simulink model "Load_Oserver"  (R2015a)
settings: Solver=ode4  StartTime=0.0  StopTime=0.1  FixedStep=1e-6  MaxStep=0.00001  MinStep=0.000001  RelTol=1e-3
libraries: powerlib x10, simulink x5, powerlib_meascontrol x3
settings Model: Creator=hp  LastModifiedBy=hp
settings SolverCC: ZeroCrossControl=DisableAll

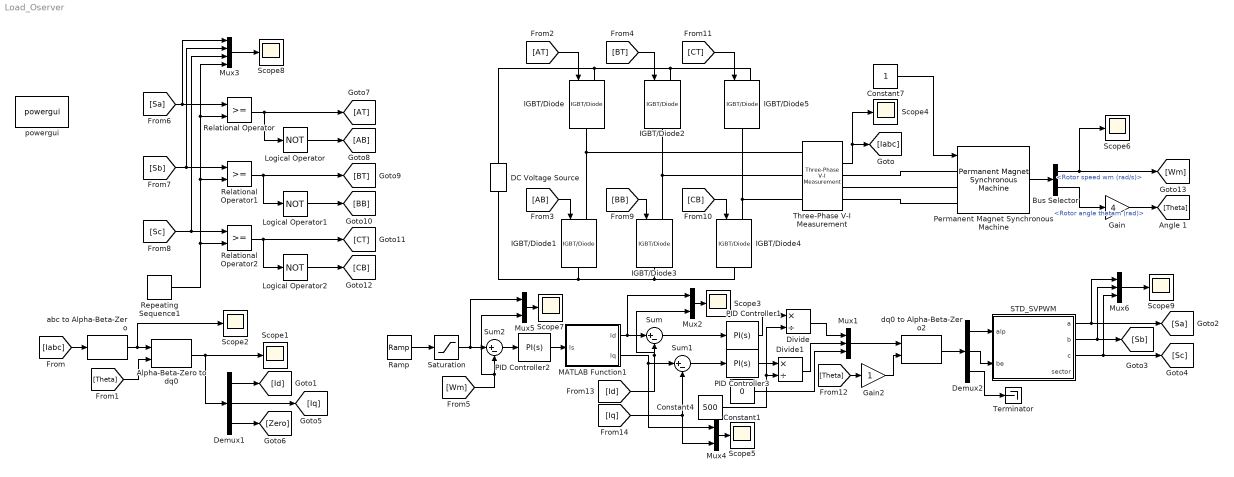
== system Load_Oserver ==
  Alpha-Beta-Zero to dq0 : powerlib_meascontrol/Transformations/Alpha-Beta-Zero to dq0  Alignment=Aligned with phase A axis
  Bus Selector : BusSelector  OutputSignals=Rotor speed wm (rad/s),Rotor angle thetam (rad)
  Constant1 : Constant  Value=0
  Constant4 : Constant  Value=500
  Constant7 : Constant
  DC Voltage Source : powerlib/Electrical Sources/DC Voltage Source  Amplitude=500  Measurements=None
  Demux1 : Demux  Outputs=3
  Demux2 : Demux  Outputs=3
  Divide : Product  Inputs=*/
  Divide1 : Product  Inputs=*/
  Gain : Gain  Gain=4
  Gain2 : Gain
  IGBT/Diode{,1..5} (6 alike) : powerlib/Power Electronics/IGBT//Diode  Ron=1e-3  Rs=1e5  Cs=inf  Measurements=off
  Logical Operator : Logic  Operator=NOT  Inputs=1  AllPortsSameDT=off  OutDataTypeStr=boolean
  Logical Operator1 : Logic  Operator=NOT  Inputs=1  AllPortsSameDT=off  OutDataTypeStr=boolean
  Logical Operator2 : Logic  Operator=NOT  Inputs=1  AllPortsSameDT=off  OutDataTypeStr=boolean
  MATLAB Function1 : MATLAB Function  TreatAsAtomicUnit=on
  Mux1 : Mux  Inputs=3
  Mux2 : Mux  Inputs=2
  Mux3 : Mux
  Mux4 : Mux  Inputs=2
  Mux5 : Mux  Inputs=2
  Mux6 : Mux  Inputs=3
  PID Controller1 : simulink/Continuous/PID Controller  Controller=PI  TimeDomain=Continuous-time  SampleTime=-1  IntegratorMethod=Forward Euler  FilterMethod=Forward Euler  Form=Parallel  UseFilter=on  ControllerParametersSource=internal  P=40  I=15000  D=0  N=100  InitialConditionSource=internal  InitialConditionForIntegrator=0  InitialConditionForFilter=0  ExternalReset=none  LimitOutput=off  UpperSaturationLimit=inf  LowerSaturationLimit=-inf  LinearizeAsGain=on  AntiWindupMode=none  Kb=1  TrackingMode=off  Kt=1  PParamMin=[]  PParamMax=[]  IParamMin=[]  IParamMax=[]  DParamMin=[]  DParamMax=[]  NParamMin=[]  NParamMax=[]  KbParamMin=[]  KbParamMax=[]  KtParamMin=[]  KtParamMax=[]  POutMin=[]  POutMax=[]  IOutMin=[]  IOutMax=[]  DOutMin=[]  DOutMax=[]  NOutMin=[]  NOutMax=[]  KbOutMin=[]  KbOutMax=[]  KtOutMin=[]  KtOutMax=[]  IntegratorOutMin=[]  IntegratorOutMax=[]  FilterOutMin=[]  FilterOutMax=[]  SumOutMin=[]  SumOutMax=[]  SumI1OutMin=[]  SumI1OutMax=[]  SumI2OutMin=[]  SumI2OutMax=[]  SumI3OutMin=[]  SumI3OutMax=[]  SumDOutMin=[]  SumDOutMax=[]  SaturationOutMin=[]  SaturationOutMax=[]  IntegratorContinuousStateAttributes=''  IntegratorStateMustResolveToSignalObject=off  IntegratorRTWStateStorageClass=Auto  FilterContinuousStateAttributes=''  FilterStateMustResolveToSignalObject=off  FilterRTWStateStorageClass=Auto  DifferentiatorICPrevScaledInput=0  DifferentiatorOutMin=[]  DifferentiatorOutMax=[]
  PID Controller2 : simulink/Continuous/PID Controller  Controller=PI  TimeDomain=Continuous-time  SampleTime=-1  IntegratorMethod=Forward Euler  FilterMethod=Forward Euler  Form=Parallel  UseFilter=on  ControllerParametersSource=internal  P=60  I=10000  D=0  N=100  InitialConditionSource=internal  InitialConditionForIntegrator=0  InitialConditionForFilter=0  ExternalReset=none  LimitOutput=off  UpperSaturationLimit=inf  LowerSaturationLimit=-inf  LinearizeAsGain=on  AntiWindupMode=none  Kb=1  TrackingMode=off  Kt=1  PParamMin=[]  PParamMax=[]  IParamMin=[]  IParamMax=[]  DParamMin=[]  DParamMax=[]  NParamMin=[]  NParamMax=[]  KbParamMin=[]  KbParamMax=[]  KtParamMin=[]  KtParamMax=[]  POutMin=[]  POutMax=[]  IOutMin=[]  IOutMax=[]  DOutMin=[]  DOutMax=[]  NOutMin=[]  NOutMax=[]  KbOutMin=[]  KbOutMax=[]  KtOutMin=[]  KtOutMax=[]  IntegratorOutMin=[]  IntegratorOutMax=[]  FilterOutMin=[]  FilterOutMax=[]  SumOutMin=[]  SumOutMax=[]  SumI1OutMin=[]  SumI1OutMax=[]  SumI2OutMin=[]  SumI2OutMax=[]  SumI3OutMin=[]  SumI3OutMax=[]  SumDOutMin=[]  SumDOutMax=[]  SaturationOutMin=[]  SaturationOutMax=[]  IntegratorContinuousStateAttributes=''  IntegratorStateMustResolveToSignalObject=off  IntegratorRTWStateStorageClass=Auto  FilterContinuousStateAttributes=''  FilterStateMustResolveToSignalObject=off  FilterRTWStateStorageClass=Auto  DifferentiatorICPrevScaledInput=0  DifferentiatorOutMin=[]  DifferentiatorOutMax=[]
  PID Controller3 : simulink/Continuous/PID Controller  Controller=PI  TimeDomain=Continuous-time  SampleTime=-1  IntegratorMethod=Forward Euler  FilterMethod=Forward Euler  Form=Parallel  UseFilter=on  ControllerParametersSource=internal  P=40  I=15000  D=0  N=100  InitialConditionSource=internal  InitialConditionForIntegrator=0  InitialConditionForFilter=0  ExternalReset=none  LimitOutput=off  UpperSaturationLimit=inf  LowerSaturationLimit=-inf  LinearizeAsGain=on  AntiWindupMode=none  Kb=1  TrackingMode=off  Kt=1  PParamMin=[]  PParamMax=[]  IParamMin=[]  IParamMax=[]  DParamMin=[]  DParamMax=[]  NParamMin=[]  NParamMax=[]  KbParamMin=[]  KbParamMax=[]  KtParamMin=[]  KtParamMax=[]  POutMin=[]  POutMax=[]  IOutMin=[]  IOutMax=[]  DOutMin=[]  DOutMax=[]  NOutMin=[]  NOutMax=[]  KbOutMin=[]  KbOutMax=[]  KtOutMin=[]  KtOutMax=[]  IntegratorOutMin=[]  IntegratorOutMax=[]  FilterOutMin=[]  FilterOutMax=[]  SumOutMin=[]  SumOutMax=[]  SumI1OutMin=[]  SumI1OutMax=[]  SumI2OutMin=[]  SumI2OutMax=[]  SumI3OutMin=[]  SumI3OutMax=[]  SumDOutMin=[]  SumDOutMax=[]  SaturationOutMin=[]  SaturationOutMax=[]  IntegratorContinuousStateAttributes=''  IntegratorStateMustResolveToSignalObject=off  IntegratorRTWStateStorageClass=Auto  FilterContinuousStateAttributes=''  FilterStateMustResolveToSignalObject=off  FilterRTWStateStorageClass=Auto  DifferentiatorICPrevScaledInput=0  DifferentiatorOutMin=[]  DifferentiatorOutMax=[]
  Permanent Magnet Synchronous Machine : powerlib/Machines/Permanent Magnet Synchronous Machine  NbPhases=3  FluxDistribution=Sinusoidal  RotorType=Salient-pole  MechanicalLoad=Torque Tm  PresetModel=No  ShowDetailedParameters=on  MeasurementBus=off  Resistance=2.07  Inductance=8.5e-3  dqInductances=[30.0e-3,2.5e-3]  La=5e-3  MachineConstant=Voltage Constant (V_peak L-L / krpm)  Flux=0.075808  VoltageCst=55  TorqueCst=0.45485  Flat=120  Mechanical=[0.00027 0.004924 4 0]  PolePairs=2  InitialConditions=[0,0, 0,0]  InitialConditions5ph=[0 0 0 0 0 0]  TsPowergui=0  TsBlock=-1  RefAngle=Aligned with phase A axis (original Park)
  Ramp : simulink/Sources/Ramp  slope=10000  start=0  X0=0
  Relational Operator : RelationalOperator  OutDataTypeStr=boolean
  Relational Operator1 : RelationalOperator  OutDataTypeStr=boolean
  Relational Operator2 : RelationalOperator  OutDataTypeStr=boolean
  Repeating Sequence1 : simulink/Sources/Repeating Sequence  rep_seq_t=[0 0.5 1]/10000  rep_seq_y=[0 1 0]
  STD_SVPWM : MATLAB Function  TreatAsAtomicUnit=on
  Saturation : Saturate  UpperLimit=300  LowerLimit=-300
  Scope{1..9} (9 alike) : Scope
      Scope1 settings: YMin=-22.5  YMax=7.5
      Scope2 settings: YMin=-1  YMax=1.75  SaveName=ScopeData2
      Scope3 settings: TimeRange=0.08752399999999999  YMin=-2  YMax=14
      Scope4 settings: YMin=-15  YMax=15  SaveName=ScopeData5
      Scope5 settings: YMin=-54  YMax=55  SaveName=ScopeData3
      Scope6 settings: YMin=-100  YMax=100  SaveName=ScopeData6
      Scope7 settings: TimeRange=0.1  YMax=500  SaveName=ScopeData4
      Scope8 settings: YMin=0  YMax=1  SaveName=ScopeData7
      Scope9 settings: YMin=0.225  YMax=0.775  SaveName=ScopeData8
  Sum : Sum  Inputs=|+-
  Sum1 : Sum  Inputs=|+-
  Sum2 : Sum  Inputs=|+-
  Terminator : Terminator
  Three-Phase V-I Measurement : powerlib/Measurements/Three-Phase V-I Measurement  VoltageMeasurement=phase-to-phase  SetLabelV=off  LabelV=Vabc  Vpu=off  VpuLL=off  CurrentMeasurement=yes  SetLabelI=off  LabelI=Iabc  Ipu=off  Pbase=100e6  Vbase=500e3  OutputType=Complex  PhasorSimulation=off  PSBequivalent=0
  abc to Alpha-Beta-Zero : powerlib_meascontrol/Transformations/abc to Alpha-Beta-Zero
  dq0 to Alpha-Beta-Zero2 : powerlib_meascontrol/Transformations/dq0 to Alpha-Beta-Zero  Alignment=Aligned with phase A axis
  powergui : powerlib/powergui  Priority=1  SimulationMode=Discrete  SolverType=Tustin/Backward Euler (TBE)  SampleTime=1e-6  frequency=60  SPID=off  DisableSnubberDevices=off  DisableRonSwitches=off  DisableVfSwitches=off  SwTol=0  DisplayEquations=off  Interpol=off  methode=off  Ts=100  FunctionMessages=off  echomessages=off  HookPort=off  EnableUseOfTLC=off  x0status=blocks  frequencyindice=0  Pbase=100e6  ErrMax=1e-4  Iterations=50  UnitsV=kV  UnitsW=MW  buscounter=0  RestoreLinks=warning  ResistiveCurrentMeasurement=off  Frange=[0:2:500]  Ylog=off  Xlog=on  ShowGrid=off  save=off  variable=ZData  structure=0  ZoomFFT=off  StartTime=0.0  cycles=1  DisplayStyle=1  fundamental=60  FreqAxis=off  MaxFrequency=1000  frequencyindicesteady=1  RmsSteady=1  display=off
  wires:
  STD_SVPWM/1(a) -> Mux6/1, [Sa]
  STD_SVPWM/2(b) -> Mux6/2, [Sb]
  STD_SVPWM/3(c) -> Mux6/3, [Sc]
  Three-Phase V-I Measurement/2 -> Scope4/1, [Iabc]
  [Iabc] -> abc to Alpha-Beta-Zero/1
  Alpha-Beta-Zero to dq0/1 -> Demux1/1, Scope1/1
  abc to Alpha-Beta-Zero/1 -> Scope2/1, Alpha-Beta-Zero to dq0/1
  [Theta] -> Alpha-Beta-Zero to dq0/2
  Demux1/1 -> [Id]
  Demux1/2 -> [Iq]
  Demux1/3 -> [Zero]
  [Sa] -> Mux3/1, Relational Operator/1
  Repeating Sequence1/1 -> Relational Operator2/2, Mux3/4, Relational Operator/2, Relational Operator1/2
  [Sb] -> Mux3/2, Relational Operator1/1
  [Sc] -> Mux3/3, Relational Operator2/1
  Relational Operator/1 -> Logical Operator/1, [AT]
  Logical Operator/1 -> [AB]
  Relational Operator1/1 -> Logical Operator1/1, [BT]
  Logical Operator1/1 -> [BB]
  Relational Operator2/1 -> Logical Operator2/1, [CT]
  Logical Operator2/1 -> [CB]
  [AT] -> IGBT/Diode/1
  [AB] -> IGBT/Diode1/1
  [BT] -> IGBT/Diode2/1
  [BB] -> IGBT/Diode3/1
  [CB] -> IGBT/Diode4/1
  [CT] -> IGBT/Diode5/1
  dq0 to Alpha-Beta-Zero2/1 -> Demux2/1
  Demux2/1 -> STD_SVPWM/1(alp)
  Demux2/2 -> STD_SVPWM/2(be)
  Demux2/3 -> Terminator/1
  [Theta] -> Gain2/1
  Gain2/1 -> dq0 to Alpha-Beta-Zero2/2
  Mux1/1 -> dq0 to Alpha-Beta-Zero2/1
  Constant1/1 -> Mux1/3
  Sum/1 -> PID Controller1/1
  Sum1/1 -> PID Controller3/1
  Mux2/1 -> Scope3/1
  [Iq] -> Mux4/2, Sum1/2
  Mux4/1 -> Scope5/1
  [Id] -> Mux2/2, Sum/2
  Constant7/1 -> Permanent Magnet Synchronous Machine/1
  Permanent Magnet Synchronous Machine/1 -> Bus Selector/1
  Bus Selector/1 -> [Wm], Scope6/1  "<Rotor speed wm (rad/s)>"
  Gain/1 -> [Theta]
  Bus Selector/2 -> Gain/1  "<Rotor angle thetam (rad)>"
  Divide/1 -> Mux1/1
  PID Controller3/1 -> Divide1/1
  Divide1/1 -> Mux1/2
  PID Controller1/1 -> Divide/1
  Constant4/1 -> Divide/2, Divide1/2
  Mux3/1 -> Scope8/1
  MATLAB Function1/1(Id) -> Mux2/1, Sum/1
  Sum2/1 -> PID Controller2/1
  Saturation/1 -> Mux5/1, Sum2/1
  Ramp/1 -> Saturation/1
  Mux5/1 -> Scope7/1
  [Wm] -> Mux5/2, Sum2/2
  Mux6/1 -> Scope9/1
  MATLAB Function1/2(Iq) -> Mux4/1, Sum1/1
  PID Controller2/1 -> MATLAB Function1/1(Is)
  connections:
  Three-Phase V-I Measurement/RConn1 -- Permanent Magnet Synchronous Machine/LConn1
  Three-Phase V-I Measurement/RConn2 -- Permanent Magnet Synchronous Machine/LConn2
  Three-Phase V-I Measurement/RConn3 -- Permanent Magnet Synchronous Machine/LConn3
  IGBT/Diode/RConn1 -- IGBT/Diode1/LConn1 -- Three-Phase V-I Measurement/LConn1
  IGBT/Diode2/RConn1 -- Three-Phase V-I Measurement/LConn2 -- IGBT/Diode3/LConn1
  IGBT/Diode5/RConn1 -- Three-Phase V-I Measurement/LConn3 -- IGBT/Diode4/LConn1
  IGBT/Diode1/RConn1 -- DC Voltage Source/LConn1 -- IGBT/Diode3/RConn1 -- IGBT/Diode4/RConn1
  IGBT/Diode/LConn1 -- DC Voltage Source/RConn1 -- IGBT/Diode2/LConn1 -- IGBT/Diode5/LConn1

== matlab function Load_Oserver/MATLAB Function1 ==
  data: Is input; Id output; Iq output
function [Id,Iq] = fcn(Is)
%#codegen
Id = (-0.3 + sqrt((0.3*0.3)+ (8*((30e-3) - (2.5e-3))*((30e-3) - (2.5e-3))*Is*Is)))/(4*((30e-3) - (2.5e-3)));
Iq = sign(Is)*sqrt((Is*Is)-(Id*Id));

== matlab function Load_Oserver/STD_SVPWM ==
  data: alp input; a output; be input; b output; c output; sector output
function [a,b,c,sector] = fcn(alp,be)
%#codegen
	sec_a=0,sec_b=0,sec_c=0;
	t_o = 0,ta = 0,tb = 0,tc = 0,tsec = 0;

    sec_a = be;										%Beta;
	sec_b = ((-be/2)+(alp*0.866));			%(-0.5*Beta+(0.866*alpha));
	sec_c = ((-be/2)-(alp*0.866));			%(-0.5*Beta-(0.866*alpha));
    
    if(sec_a>=0)
       if(sec_b>=0)
       												%	sector 1
    		t_o = (1 - (sec_a+sec_b))/2;							%	t_1 = sec_b, t_2 =sec_a
    		ta = sec_a+sec_b+(t_o);
    		tb  = sec_a+(t_o);
    		tc  = (t_o);
            tsec = 1;
       else
            if(sec_c>=0)												%	sector 3
        		t_o = (1 - (sec_a+sec_c))/2;						%	t_1 = sec_a, t_2 =sec_c
        		ta = (t_o);
        		tb = sec_a+sec_c+(t_o);
        		tc = sec_c+(t_o);
                tsec = 3;
            else												%	sector 2
        		t_o = (1 + (sec_c+sec_b))/2;					%	t_1 = -sec_c, t_2 =-sec_b
        		ta = -sec_c+(t_o);
        		tb = -(sec_c+sec_b)+(t_o);
        		tc = (t_o);
                tsec = 2;
            end
       end
    else
       if(sec_b>=0)
           if(sec_c>=0)                                                  %	sector 5
        		t_o = (1 - (sec_c+sec_b))/2; 				%	t_1 = sec_c, t_2 =sec_b
        		ta = sec_b+(t_o);
        		tb = (t_o);
        		tc = sec_c+sec_b+(t_o);
                tsec = 5;
           else                                                  %	sector 6
        		t_o = (1 + (sec_a+sec_c))/2; 				%	t_1 = -sec_a, t_2 =-sec_c
        		ta = -(sec_a+sec_c)+(t_o);
        		tb = (t_o);
        		tc = -sec_a+(t_o);
                tsec = 6;
           end
       else
            if(sec_c>=0)                                      %	sector 4
        		t_o = (1 + (sec_a+sec_b))/2;			%	t_1 = -sec_b, t_2 =-sec_a
        		ta = (t_o);
        		tb = -sec_b+(t_o);
        		tc = -(sec_a+sec_b)+(t_o);
                tsec = 4;
            end
       end
    end
a = ta;
b = tb;
c = tc;
sector = tsec;
